simulink model "ensayos_pll"  (R2024a)
settings: Solver=FixedStepAuto  StartTime=0.0  StopTime=1  RelTol=1e-3
values from neighbouring files (symbols this model uses):
  start_frec = 50    [ensayo_pll.m]
  step_time = 0.5    [ensayo_pll.m]    (also in simulacion.m = 10)
libraries: spsGroundLib x1, spsPLL3phLib x1, spsThreePhaseProgrammableVoltageSourceLib x1, spsThreePhaseVIMeasurementLib x1, sps_lib x1
settings Model: Creator=sebar  LastModifiedBy=sebar

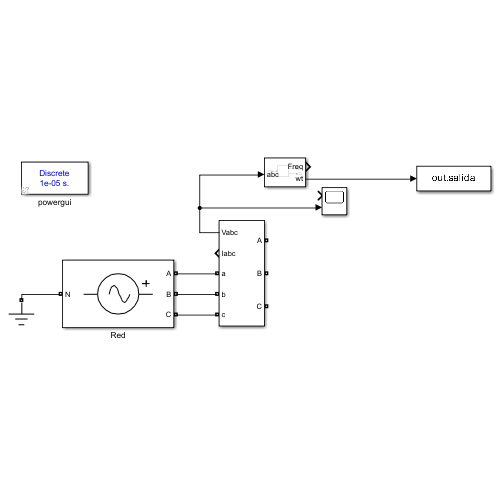
[thumbnail: Simulink's stored preview of the top-level diagram]
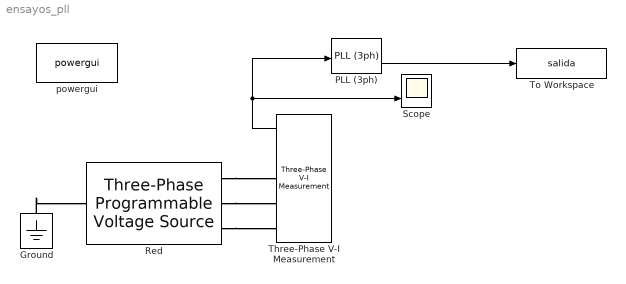
== system ensayos_pll ==
  Ground : spsGroundLib/Ground  LConnTagsString=a
  PLL (3ph) : spsPLL3phLib/PLL (3ph)  Fmin=45  Par_Init=[0, 50]  ParK=[300, 4000, 1]  TcD=1e-4  MaxRateChangeFreq=50  FilterCutOffFreq=50  Ts=0  AGC=on
  Red : spsThreePhaseProgrammableVoltageSourceLib/Three-Phase Programmable Voltage Source  PositiveSequence="[28*sqrt(3)  0 start_frec]"  VariationEntity=Phase  VariationType=Table of time-amplitude pairs  VariationTypeAlt=Step  VariationStep=step_size  VariationRate=10  VariationMagnitude=0.3  VariationFrequency=2  VariationTiming=[step_time 1e10]  VariationPhaseA=off  Amplitudes=[1 0.8 1.2 1.0]  TimeValues=[0 0.1 0.15 0.2]  HarmonicGeneration=off  HarmonicA=[3 0.2 -25 0]  HarmonicB=[2 0.15 35 2]  Timing="[0.05  3]"  BusType=swing  Pref=0  Qref=0  Qmin=-inf  Qmax=inf
  Scope : Scope  NumInputPorts=2
  Three-Phase V-I Measurement : spsThreePhaseVIMeasurementLib/Three-Phase V-I Measurement  VoltageMeasurement=phase-to-ground  SetLabelV=off  LabelV=Vabc  Vpu=off  VpuLL=off  CurrentMeasurement=yes  SetLabelI=off  LabelI=Iabc  Ipu=off  Pbase=100e6  Vbase=500e3  OutputType=Complex  PhasorSimulation=off  PSBequivalent=0
  To Workspace : ToWorkspace  VariableName=salida  SampleTime=-1
  powergui : sps_lib/powergui  Priority=1  SimulationMode=Discrete  SampleTime=1e-5  frequency=60  Iterations=50  frequencyindice=50  Pbase=100e6  ErrMax=1e-4  UnitsV=kV  UnitsW=MW  buscounter=0  FunctionMessages=off  echomessages=off  EnableUseOfTLC=off  CurrentSourceSwitches=off  DisableSnubberDevices=off  DisableRonSwitches=off  DisableVfSwitches=off  DisplayEquations=off  AutomaticDiscreteSolvers=off  SolverType=Tustin/Backward Euler (TBE)  Interpol=off  ExternalGateDelay=off  methode=off  Ts=100  x0status=blocks  SPID=on  SwTol=0  HookPort=off  NonlinearTolerance=1e-4  nMaxIteration=100  ContinueOnMaxIteration=off  RestoreLinks=warning  ResistiveCurrentMeasurement=off  Frange=[0:2:500]  Ylog=off  Xlog=on  ShowGrid=off  save=off  variable=ZData  structure=0  ZoomFFT=off  StartTime=0.0  cycles=1  DisplayStyle=1  fundamental=60  FreqAxis=off  MaxFrequency=1000  frequencyindicesteady=1  RmsSteady=1  display=off
  wires:
  Three-Phase V-I Measurement/1 -> PLL (3ph)/1, Scope/2
  PLL (3ph)/2 -> To Workspace/1
  connections:
  Red/RConn1 -- Three-Phase V-I Measurement/RConn1
  Red/RConn2 -- Three-Phase V-I Measurement/RConn2
  Red/RConn3 -- Three-Phase V-I Measurement/RConn3
  Ground/LConn1 -- Red/LConn1
